simulink model "MGS_linearizedInvertedPendulum_Cart_Simplified_mdl"  (R2022b)
settings: Solver=ode4  StartTime=0.0  StopTime=25  FixedStep=.001  RelTol=1e-3
undefined symbols (not defined in the file): F, G, P_0
settings Model: Creator=mo780715  LastModifiedBy=mohammadodeh

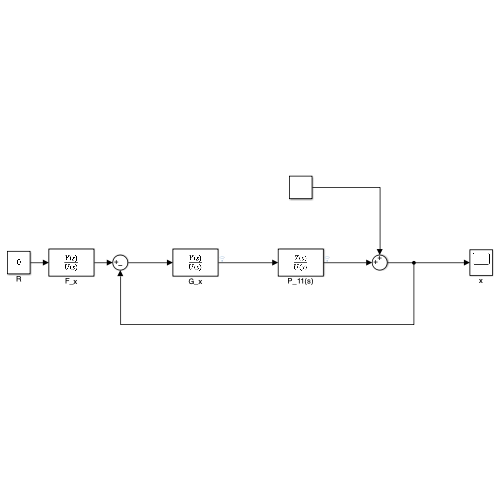
[thumbnail: Simulink's stored preview of the top-level diagram]
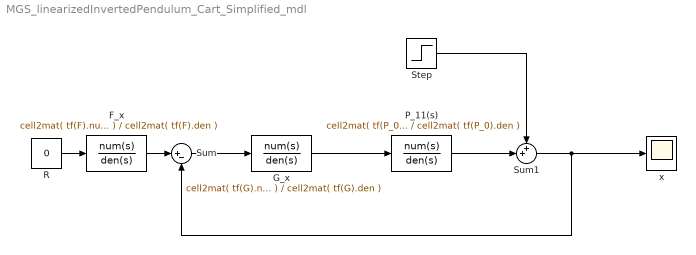
== system MGS_linearizedInvertedPendulum_Cart_Simplified_mdl ==
  F_x : TransferFcn  Numerator=cell2mat( tf(F).num )  Denominator=cell2mat( tf(F).den )  ContinuousStateAttributes='x'
  G_x : TransferFcn  Numerator=cell2mat( tf(G).num )  Denominator=cell2mat( tf(G).den )  ContinuousStateAttributes='x'
  P_11(s) : TransferFcn  Numerator=cell2mat( tf(P_0).num )  Denominator=cell2mat( tf(P_0).den )  ContinuousStateAttributes='x'
  R : Constant  Value=0
  Step : Step  SampleTime=0
  Sum : Sum  Inputs=|+-
  Sum1 : Sum  Inputs=++|
  x : Scope
  wires:
  R/1 -> F_x/1
  F_x/1 -> Sum/1
  Sum/1 -> G_x/1
  G_x/1 -> P_11(s)/1
  P_11(s)/1 -> Sum1/2
  Sum1/1 -> Sum/2, x/1
  Step/1 -> Sum1/1
